simulink model "SimulationOfFurutaL2"  (R2017a)
settings: Solver=ode5  StartTime=0.0  StopTime=20  FixedStep=0.01  RelTol=1e-3
values from neighbouring files (symbols this model uses):
  b10 = 6.05e-3    (= 0.00605)    [FurutaConstants.m]
  b20 = 5.52e-04    (= 0.000552)    [FurutaConstants.m]
  g0 = 9.81    [FurutaConstants.m]
  I2y0 = 0.2937e-3    (= 0.0002937)    [FurutaConstants.m]
  I2z0 = 0.0051e-3    (= 5.1e-06)    [FurutaConstants.m]
  Ixz20 = -0.0131e-3    (= -1.31e-05)    [FurutaConstants.m]
  k10 = (I2y0 + I1z0 + L10^2*m20+l10^2*m10+l20^2*m20)/2    (= 0.00399493504648)    [FurutaConstants.m]
  k20 = (I2x0+l20^2*m20)/2    (= 0.000230092732776)    [FurutaConstants.m]
  kt0 = 0.122326    [FurutaConstants.m]
  L10 = 230.45e-3    (= 0.23045)    [FurutaConstants.m]
  l20 = 58.18e-3    (= 0.05818)    [FurutaConstants.m]
  L20 = 239.73e-3    (= 0.23973)    [FurutaConstants.m]
  m20 = 0.04948    [FurutaConstants.m]
  Rm0 = 12.38    [FurutaConstants.m]
settings Model: Creator=felip  LastModifiedBy=felip

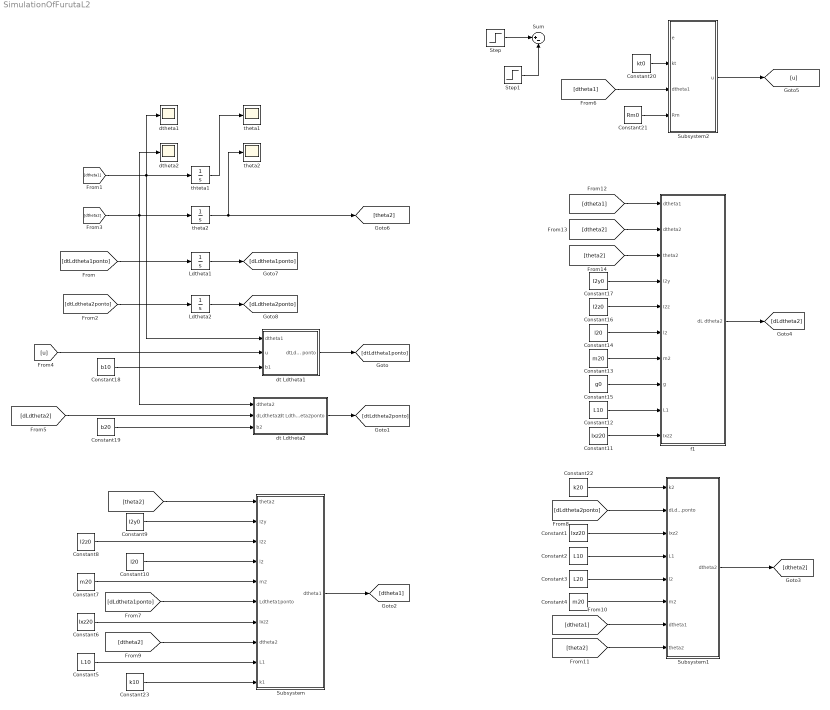
== system SimulationOfFurutaL2 ==
  Constant1 : Constant  Value=Ixz20
  Constant10 : Constant  Value=l20
  Constant11 : Constant  Value=Ixz20
  Constant12 : Constant  Value=L10
  Constant13 : Constant  Value=m20
  Constant14 : Constant  Value=l20
  Constant15 : Constant  Value=g0
  Constant16 : Constant  Value=I2z0
  Constant17 : Constant  Value=I2y0
  Constant18 : Constant  Value=b10
  Constant19 : Constant  Value=b20
  Constant2 : Constant  Value=L10
  Constant20 : Constant  Value=kt0
  Constant21 : Constant  Value=Rm0
  Constant22 : Constant  Value=k20
  Constant23 : Constant  Value=k10
  Constant3 : Constant  Value=L20
  Constant4 : Constant  Value=m20
  Constant5 : Constant  Value=L10
  Constant6 : Constant  Value=Ixz20
  Constant7 : Constant  Value=m20
  Constant8 : Constant  Value=I2z0
  Constant9 : Constant  Value=I2y0
  Ldtheta1 : Integrator
  Ldtheta2 : Integrator
  Step : Step  Time=0  After=5  SampleTime=0
  Step1 : Step  Time=1/5  After=5  SampleTime=0
  Subsystem : Subsystem
  Subsystem1 : Subsystem
  Subsystem2 : Subsystem
  Sum : Sum  Inputs=|+-
  dt Ldtheta1 : Subsystem
  dt Ldtheta2 : Subsystem
  dtheta1 : Scope
  "dtheta2 " : Scope
  f1 : Subsystem
  theta1 : Scope
  theta2 : Integrator  InitialCondition=pi/2
  "theta2 " : Scope
  thteta1 : Integrator
  wires:
  [dtheta1] -> thteta1/1, dtheta1/1, dt Ldtheta1/1(dtheta1)
  [u] -> dt Ldtheta1/2(u)
  Constant18/1 -> dt Ldtheta1/3(b1)
  dt Ldtheta1/1("dtLdtheta1 ponto ") -> [dtLdtheta1ponto]
  [dtLdtheta1ponto] -> Ldtheta1/1
  [dtLdtheta2ponto] -> Ldtheta2/1
  [dtheta2] -> "dtheta2 "/1, theta2/1, dt Ldtheta2/1("dtheta2 ")
  Constant19/1 -> dt Ldtheta2/3(b2)
  dt Ldtheta2/1(dt Ldtheta2ponto) -> [dtLdtheta2ponto]
  [dLdtheta2] -> dt Ldtheta2/2("dLdtheta2 ")
  Subsystem/1("dtheta1 ") -> [dtheta1]
  Subsystem1/1(dtheta2) -> [dtheta2]
  f1/1("dL dtheta2 ") -> [dLdtheta2]
  thteta1/1 -> theta1/1
  Ldtheta1/1 -> [dLdtheta1ponto]
  Ldtheta2/1 -> [dLdtheta2ponto]
  [theta2] -> Subsystem/1(theta2)
  [dLdtheta1ponto] -> Subsystem/6("Ldtheta1ponto ")
  [dLdtheta2ponto] -> Subsystem1/2(dLdtheta2ponto)
  [dtheta2] -> Subsystem/8(dtheta2)
  [dtheta1] -> Subsystem1/7("dtheta1 ")
  [theta2] -> Subsystem1/8(theta2)
  [dtheta2] -> f1/2(dtheta2)
  [dtheta1] -> f1/1(dtheta1)
  [theta2] -> f1/3(theta2)
  Constant6/1 -> Subsystem/7(Ixz2)
  Constant13/1 -> f1/7("m2 ")
  Constant15/1 -> f1/8(g)
  Constant1/1 -> Subsystem1/3(Ixz2)
  Constant2/1 -> Subsystem1/4(L1)
  Subsystem2/1("u ") -> [u]
  Constant20/1 -> Subsystem2/2(kt)
  Constant21/1 -> Subsystem2/4(Rm)
  [dtheta1] -> Subsystem2/3(dtheta1)
  Constant22/1 -> Subsystem1/1(k2)
  Constant3/1 -> Subsystem1/5(l2)
  Constant4/1 -> Subsystem1/6(m2)
  Constant5/1 -> Subsystem/9(L1)
  Constant7/1 -> Subsystem/5("m2 ")
  Constant10/1 -> Subsystem/4("l2 ")
  Constant8/1 -> Subsystem/3("I2z ")
  Constant9/1 -> Subsystem/2("I2y ")
  Constant11/1 -> f1/10(Ixz2)
  Constant12/1 -> f1/9(L1)
  Constant14/1 -> f1/6(l2)
  Constant16/1 -> f1/5(I2z)
  Constant17/1 -> f1/4("I2y ")
  Constant23/1 -> Subsystem/10("k1 ")
  Step1/1 -> Sum/2
  Step/1 -> Sum/1
  theta2/1 -> [theta2], "theta2 "/1

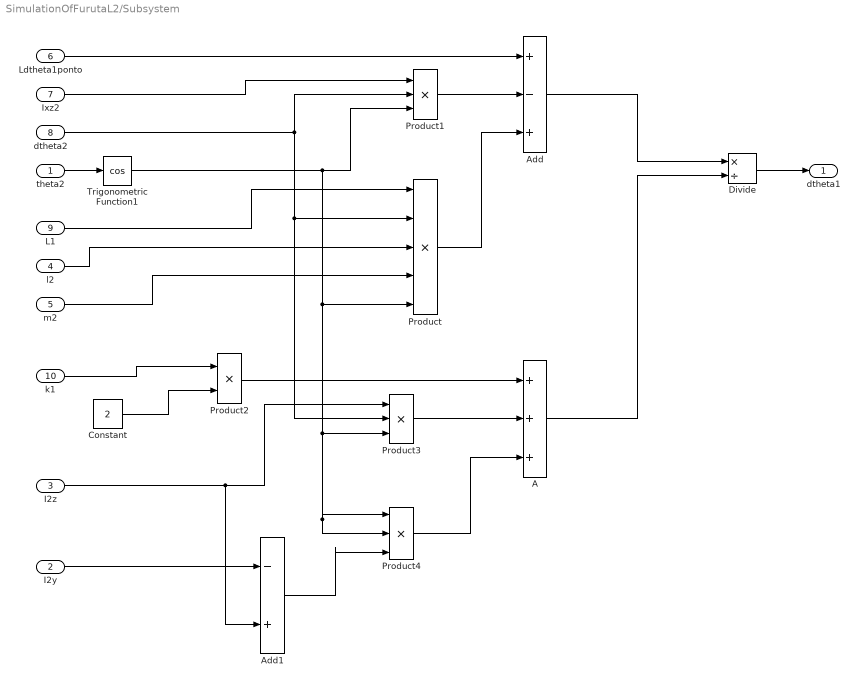
== system SimulationOfFurutaL2/Subsystem ==
  theta2 : Inport
  "I2y " : Inport  Port=2
  "I2z " : Inport  Port=3
  "l2 " : Inport  Port=4
  "m2 " : Inport  Port=5
  "Ldtheta1ponto " : Inport  Port=6
  Ixz2 : Inport  Port=7
  dtheta2 : Inport  Port=8
  L1 : Inport  Port=9
  "k1 " : Inport  Port=10
  A : Sum  Inputs=+++
  Add : Sum  Inputs=+-+
  "Add1 " : Sum  Inputs=-+
  Constant : Constant  Value=2
  Divide : Product  Inputs=*/
  Product : Product  Inputs=5
  Product1 : Product  Inputs=3
  Product2 : Product
  Product3 : Product  Inputs=3
  Product4 : Product  Inputs=3
  Trigonometric Function1 : Trigonometry  Operator=cos
  "dtheta1 " : Outport
  wires:
  Divide/1 -> "dtheta1 "/1
  "Ldtheta1ponto "/1 -> Add/1
  Product1/1 -> Add/2
  Ixz2/1 -> Product1/1
  dtheta2/1 -> Product3/2, Product/2, Product1/2
  theta2/1 -> Trigonometric Function1/1
  Trigonometric Function1/1 -> Product/5, Product4/1, Product4/2, Product3/3, Product1/3
  Product/1 -> Add/3
  L1/1 -> Product/1
  "l2 "/1 -> Product/3
  "m2 "/1 -> Product/4
  Add/1 -> Divide/1
  Constant/1 -> Product2/2
  "k1 "/1 -> Product2/1
  Product2/1 -> A/1
  Product3/1 -> A/2
  "I2z "/1 -> "Add1 "/2, Product3/1
  "Add1 "/1 -> Product4/3
  "I2y "/1 -> "Add1 "/1
  Product4/1 -> A/3
  A/1 -> Divide/2

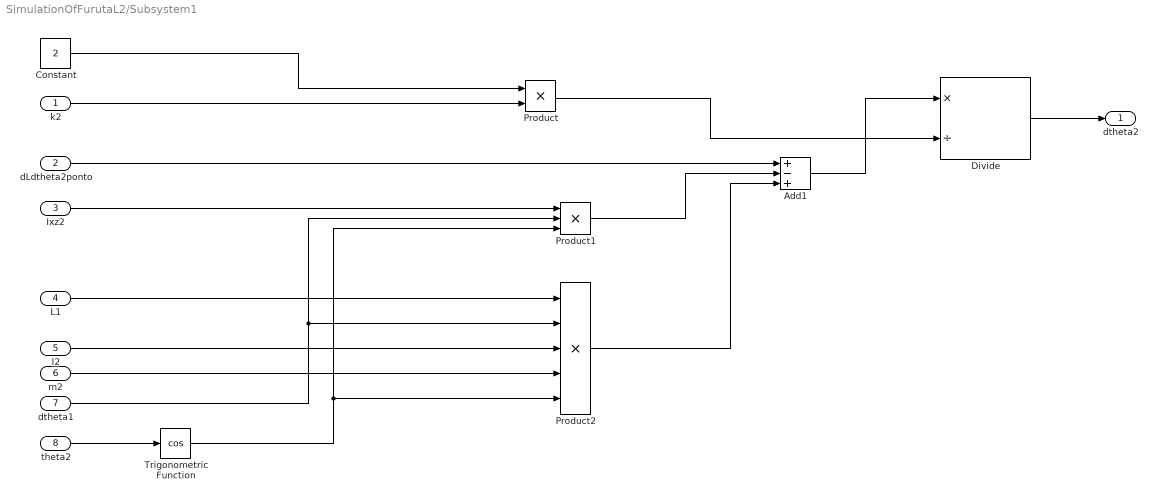
== system SimulationOfFurutaL2/Subsystem1 ==
  k2 : Inport
  dLdtheta2ponto : Inport  Port=2
  Ixz2 : Inport  Port=3
  L1 : Inport  Port=4
  l2 : Inport  Port=5
  m2 : Inport  Port=6
  "dtheta1 " : Inport  Port=7
  theta2 : Inport  Port=8
  Add1 : Sum  Inputs=+-+
  Constant : Constant  Value=2
  Divide : Product  Inputs=*/
  Product : Product
  Product1 : Product  Inputs=3
  Product2 : Product  Inputs=5
  Trigonometric Function : Trigonometry  Operator=cos
  dtheta2 : Outport
  wires:
  Divide/1 -> dtheta2/1
  Constant/1 -> Product/1
  k2/1 -> Product/2
  Product/1 -> Divide/2
  Add1/1 -> Divide/1
  dLdtheta2ponto/1 -> Add1/1
  theta2/1 -> Trigonometric Function/1
  Product1/1 -> Add1/2
  Ixz2/1 -> Product1/1
  "dtheta1 "/1 -> Product1/2, Product2/2
  Trigonometric Function/1 -> Product2/5, Product1/3
  L1/1 -> Product2/1
  l2/1 -> Product2/3
  m2/1 -> Product2/4
  Product2/1 -> Add1/3

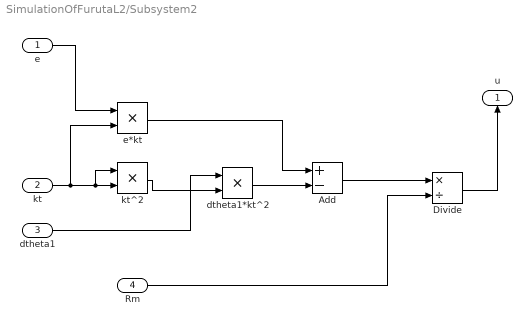
== system SimulationOfFurutaL2/Subsystem2 ==
  e : Inport
  kt : Inport  Port=2
  dtheta1 : Inport  Port=3
  Rm : Inport  Port=4
  Add : Sum  Inputs=+-
  Divide : Product  Inputs=*/
  dtheta1*kt^2 : Product
  e*kt : Product
  kt^2 : Product
  "u " : Outport
  wires:
  Divide/1 -> "u "/1
  kt/1 -> e*kt/2, kt^2/1, kt^2/2
  kt^2/1 -> dtheta1*kt^2/2
  dtheta1/1 -> dtheta1*kt^2/1
  dtheta1*kt^2/1 -> Add/2
  e/1 -> e*kt/1
  e*kt/1 -> Add/1
  Add/1 -> Divide/1
  Rm/1 -> Divide/2

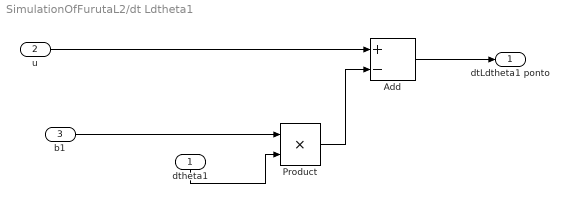
== system SimulationOfFurutaL2/dt Ldtheta1 ==
  dtheta1 : Inport
  u : Inport  Port=2
  b1 : Inport  Port=3
  Add : Sum  Inputs=+-
  Product : Product
  "dtLdtheta1 ponto " : Outport
  wires:
  Product/1 -> Add/2
  dtheta1/1 -> Product/2
  b1/1 -> Product/1
  u/1 -> Add/1
  Add/1 -> "dtLdtheta1 ponto "/1

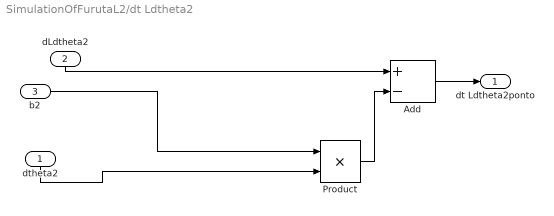
== system SimulationOfFurutaL2/dt Ldtheta2 ==
  "dtheta2 " : Inport
  "dLdtheta2 " : Inport  Port=2
  b2 : Inport  Port=3
  Add : Sum  Inputs=+-
  Product : Product
  dt Ldtheta2ponto : Outport
  wires:
  Product/1 -> Add/2
  "dtheta2 "/1 -> Product/2
  "dLdtheta2 "/1 -> Add/1
  Add/1 -> dt Ldtheta2ponto/1
  b2/1 -> Product/1

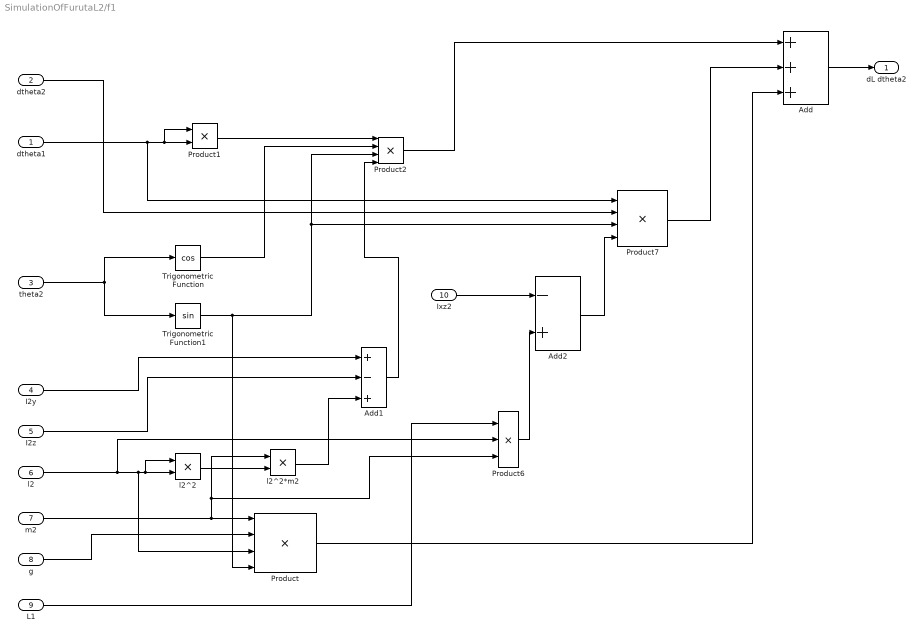
== system SimulationOfFurutaL2/f1 ==
  dtheta1 : Inport
  dtheta2 : Inport  Port=2
  theta2 : Inport  Port=3
  "I2y " : Inport  Port=4
  I2z : Inport  Port=5
  l2 : Inport  Port=6
  "m2 " : Inport  Port=7
  g : Inport  Port=8
  L1 : Inport  Port=9
  Ixz2 : Inport  Port=10
  Add : Sum  Inputs=+++
  Add1 : Sum  Inputs=+-+
  Add2 : Sum  Inputs=-+
  Product : Product  Inputs=4
  Product1 : Product
  Product2 : Product  Inputs=4
  Product6 : Product  Inputs=3
  Product7 : Product  Inputs=4
  Trigonometric Function : Trigonometry  Operator=cos
  Trigonometric Function1 : Trigonometry
  l2^2 : Product
  l2^2*m2 : Product
  "dL dtheta2 " : Outport
  wires:
  theta2/1 -> Trigonometric Function1/1, Trigonometric Function/1
  Add/1 -> "dL dtheta2 "/1
  Trigonometric Function1/1 -> Product/4, Product7/3, Product2/3
  l2/1 -> Product6/2, l2^2/1, l2^2/2, Product/3
  g/1 -> Product/2
  "m2 "/1 -> Product6/3, l2^2*m2/1, Product/1
  Product/1 -> Add/3
  dtheta1/1 -> Product7/1, Product1/1, Product1/2
  Product1/1 -> Product2/1
  Trigonometric Function/1 -> Product2/2
  Add1/1 -> Product2/4
  "I2y "/1 -> Add1/1
  I2z/1 -> Add1/2
  l2^2/1 -> l2^2*m2/2
  l2^2*m2/1 -> Add1/3
  Product2/1 -> Add/1
  Add2/1 -> Product7/4
  Product7/1 -> Add/2
  Product6/1 -> Add2/2
  L1/1 -> Product6/1
  Ixz2/1 -> Add2/1
  dtheta2/1 -> Product7/2
